simulink model "testLQG"  (R2023b)
settings: Solver=VariableStepAuto  StartTime=0.0  StopTime=1000  RelTol=1e-3
values from neighbouring files (symbols this model uses):
  Ts = 1    [CEFASSID.m]    (also in analyticModel.m = mean(time(2:end,1)-time(1:end-1,1)); cefasModel.m = mean(time(2:end,1)-time(1:end-1,1)); cefasRL_.m = 1.2273; dynamic.m = 0.1)
undefined symbols (not defined in the file or in its folder): Discrete, K, Time
libraries: ctrlSharedLib x1, simulink x1
settings Model: Creator=Anish Sebastian  LastModifiedBy=Golam Jaman

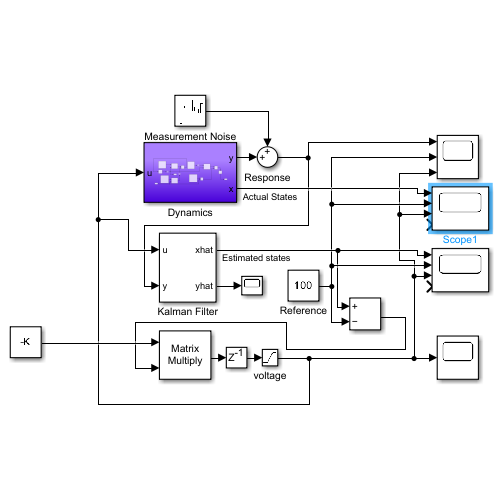
[thumbnail: Simulink's stored preview of the top-level diagram]
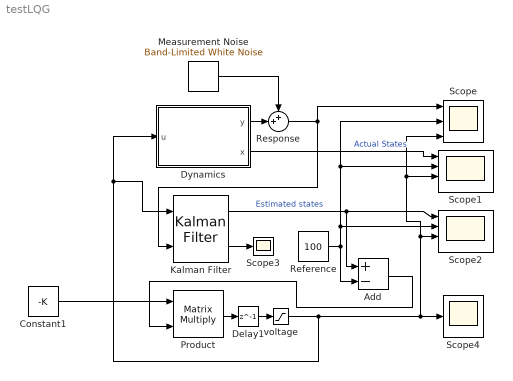
== system testLQG ==
  Add : Sum  Inputs=+-
  Constant1 : Constant  Value=-K  SampleTime=Ts
  Delay1 : Delay  DelayLength=1  InitialCondition=0
  Dynamics : Subsystem
  Kalman Filter : ctrlSharedLib/Kalman Filter  TimeDomain=Discrete-Time  UseCurrentEstimator=on  ModelSource=LTI State-Space Variable  ModelSourceVariable=test_ss  A=0.95  B=1  C=1  D=0  NumberOfStates=4  NumberOfInputs=1  NumberOfOutputs=1  InitialEstimateSource=Dialog  X0=[0]'  P0=10  UseK=off  UseGH=off  NumberOfProcessNoiseInputs=1  G=1  TimeInvariantG=on  H=0  TimeInvariantH=on  Q=0.05  TimeInvariantQ=on  R=1  TimeInvariantR=on  N=0  TimeInvariantN=on  AddInputPort=on  AddEnablePort=off  OutputEstimatedY=on  OutputP=off  Ts=-1
  Measurement Noise : simulink/Sources/Band-Limited White Noise  Cov=[0.0001]  Ts=Ts  seed=[23341]
  Product : Product  Multiplication=Matrix(*)
  Reference : Constant  Value=100  SampleTime=Ts
  Response : Sum  Inputs=++|
  Scope : Scope  NumInputPorts=3
  Scope1 : Scope  NumInputPorts=4
  Scope2 : Scope  NumInputPorts=4
  Scope3 : Scope
  Scope4 : Scope
  voltage : Saturate  UpperLimit=10  LowerLimit=0
  wires:
  Delay1/1 -> voltage/1
  Response/1 -> Kalman Filter/2, Scope/1
  Kalman Filter/2 -> Scope3/1
  Constant1/1 -> Product/1
  Add/1 -> Product/2
  Product/1 -> Delay1/1
  Measurement Noise/1 -> Response/1
  Dynamics/1(y) -> Response/2
  Kalman Filter/1 -> Add/1, Scope2/1  "Estimated states"
  Dynamics/2(x) -> Scope1/1  "Actual States"
  voltage/1 -> Kalman Filter/1, Dynamics/1(u), Scope/3, Scope1/3, Scope2/3, Scope4/1
  Reference/1 -> Scope/2, Scope1/2, Scope2/2, Add/2

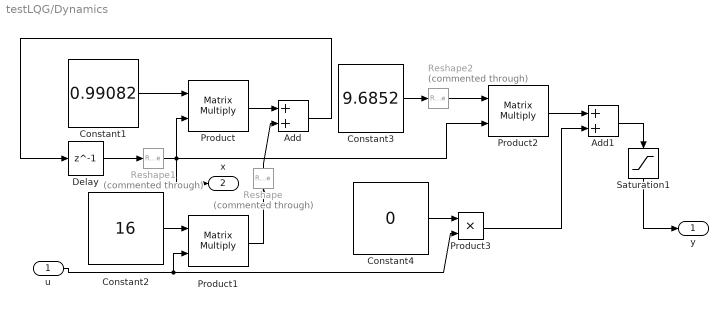
== system testLQG/Dynamics ==
  u : Inport
  Add : Sum
  Add1 : Sum
  Constant1 : Constant  Value=0.99082  SampleTime=Ts
  Constant2 : Constant  Value=16  SampleTime=Ts
  Constant3 : Constant  Value=9.6852  SampleTime=Ts
  Constant4 : Constant  Value=0  SampleTime=Ts
  Delay : Delay  DelayLength=1  InitialCondition=[0]'
  Product : Product  Multiplication=Matrix(*)
  Product1 : Product  Multiplication=Matrix(*)
  Product2 : Product  Multiplication=Matrix(*)
  Product3 : Product
  Reshape : Reshape  Commented=through  OutputDimensionality=Customize  OutputDimensions=[2,1]
  Reshape1 : Reshape  Commented=through  OutputDimensionality=Customize  OutputDimensions=[2,1]
  Reshape2 : Reshape  Commented=through  OutputDimensionality=Customize  OutputDimensions=[1,2]
  Saturation1 : Saturate  UpperLimit=inf  LowerLimit=0
  y : Outport
  x : Outport  Port=2
  wires:
  Product/1 -> Add/1
  Constant3/1 -> Reshape2/1
  Saturation1/1 -> y/1
  Constant1/1 -> Product/1
  Reshape1/1 -> Product/2, Product2/2, x/1
  Product1/1 -> Reshape/1
  Product2/1 -> Add1/1
  Reshape/1 -> Add/2
  Add/1 -> Delay/1
  Product3/1 -> Add1/2
  Constant4/1 -> Product3/1
  Reshape2/1 -> Product2/1
  Add1/1 -> Saturation1/1
  Constant2/1 -> Product1/1
  u/1 -> Product1/2, Product3/2
  Delay/1 -> Reshape1/1
